simulink model "Controller"  (R2020a)
settings: Solver=FixedStepDiscrete  StartTime=0.0  StopTime=inf  FixedStep=Ts  RelTol=1e-3
values from neighbouring files (symbols this model uses):
  driver_decel = 4.0    (= 4)    [helperLFSetUp.m]
  FB_decel = 9.8    [helperLFSetUp.m]
  Fyf1 = zeros(1,57)    [FyfLookup05.m]
  headwayOffset = 3.7    [helperLFSetUp.m]
  m = 2272    [FyfLookup05.m]    (also in helperLFSetUp.m)
  max_dc = -10    [helperLFSetUp.m]
  PB1_decel = 3.8    [helperLFSetUp.m]
  PB2_decel = 5.3    [helperLFSetUp.m]
  posSelector = [1,0,0,0,0,0; 0,0,1,0,0,0]    [helperLFSetUp.m]
  PredictionHorizon = 30    [helperLFSetUp.m]
  PredictionHorizon1 = 60    [helperLFSetUp.m]
  SlipAngle1 = -SlipAngle1    [FyfLookup05.m]
  time_gap = 1.5    [helperLFSetUp.m]
  timeMargin = 0    [helperLFSetUp.m]
  timeToReact = 1.2    [helperLFSetUp.m]
  Ts = 0.1    [helperLFSetUp.m]
libraries: drivinglib x4, simulink x2, mpcadaslib x1, mpclib x1, simulink_extras x1
(part 1 of 2)
settings Model: Creator=The MathWorks, Inc.  LastModifiedBy=dekunw
settings DataIOCC: SaveOutput=off  SaveTime=off  ReturnWorkspaceOutputs=off
settings OptimizationCC: DefaultParameterBehavior=Inlined  DefaultUnderspecifiedDataType=single  EnhancedBackFolding=on  PassReuseOutputArgsAs=Individual arguments  ZeroExternalMemoryAtStartup=off  ZeroInternalMemoryAtStartup=off  OptimizeBlockOrder=speed  DifferentSizesBufferReuse=on  OptimizationCustomize=off  EfficientTunableParamExpr=on
settings DebuggingCC: ParameterPrecisionLossMsg=none  ParameterTunabilityLossMsg=error  PregeneratedLibrarySubsystemCodeDiagnostic=none  ArithmeticOperatorsInVariantConditions=warning
settings HardwareCC: ProdLongLongMode=on
settings SFSimCC: SimUseLocalCustomCode=off  MATLABDynamicMemAlloc=off  CustomCodeUndefinedFunction=UseInterfaceOnly
settings RTWCC: SystemTargetFile=ert.tlc  TemplateMakefile=ert_default_tmf  GenerateReport=on  RTWUseLocalCustomCode=off  BuildConfiguration=Faster Runs  IncludeHyperlinkInReport=on  LaunchReport=on  TargetLang=C++  GenerateTraceInfo=on  GenerateTraceReport=on  GenerateTraceReportSl=on  GenerateTraceReportSf=on  GenerateTraceReportEml=on
settings CodeAppCC: ForceParamTrailComments=on  IgnoreCustomStorageClasses=off  MaxIdLength=63  OperatorAnnotations=on  SimulinkDataObjDesc=on  SFDataObjDesc=on  CustomSymbolStrFcn=$N$M$F  InsertBlockDesc=on
settings ERTTargetCC: TargetLangStandard=C++03 (ISO)  GenerateSampleERTMain=on  MultiInstanceERTCode=on  CodeInterfacePackaging=C++ class  InlinedParameterPlacement=NonHierarchical  RootIOFormat=Structure reference  ERTCustomFileTemplate=example_file_process.tlc

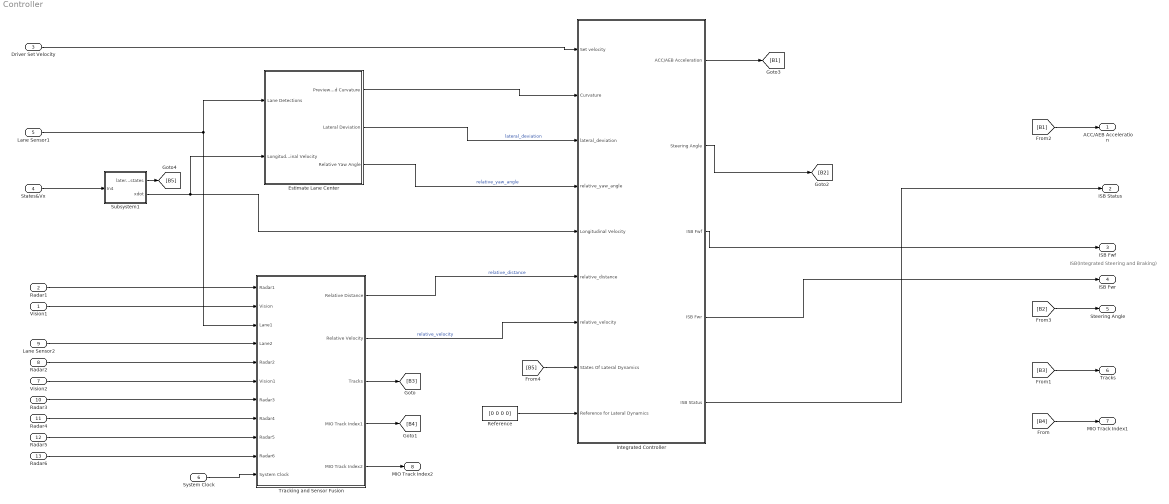
== system Controller ==
  note: ISB(Integrated Steering and Braking)
  Vision1 : Inport  OutDataTypeStr=Bus: BusVision  PortDimensions=[1 1]  BusOutputAsStruct=on
  Radar1 : Inport  Port=2  OutDataTypeStr=Bus: BusRadar  PortDimensions=[1 1]  BusOutputAsStruct=on
  Driver Set Velocity : Inport  Port=3
  States&Vx : Inport  Port=4  OutDataTypeStr=double  Unit=m/s
  Lane Sensor1 : Inport  Port=5  OutDataTypeStr=Bus: LaneSensor  PortDimensions=[1 1]
  System Clock : Inport  Port=6  OutDataTypeStr=double  PortDimensions=[1 1]
  Vision2 : Inport  Port=7  OutDataTypeStr=Bus: BusVision  PortDimensions=[1 1]  BusOutputAsStruct=on
  Radar2 : Inport  Port=8  OutDataTypeStr=Bus: BusRadar  PortDimensions=[1 1]  BusOutputAsStruct=on
  Lane Sensor2 : Inport  Port=9  OutDataTypeStr=Bus: LaneSensor  PortDimensions=[1 1]
  Radar3 : Inport  Port=10  OutDataTypeStr=Bus: BusRadar  PortDimensions=[1 1]  BusOutputAsStruct=on
  Radar4 : Inport  Port=11  OutDataTypeStr=Bus: BusRadar  PortDimensions=[1 1]  BusOutputAsStruct=on
  Radar5 : Inport  Port=12  OutDataTypeStr=Bus: BusRadar  PortDimensions=[1 1]  BusOutputAsStruct=on
  Radar6 : Inport  Port=13  OutDataTypeStr=Bus: BusRadar  PortDimensions=[1 1]  BusOutputAsStruct=on
  Estimate Lane Center : Subsystem  TreatAsAtomicUnit=on  VariantControl=v2
      settings: RTWFileNameOpts=Use function name
  Integrated Controller : Subsystem
  Reference : Constant  Value=[0 0 0 0]
  Subsystem1 : Subsystem
  Tracking and Sensor Fusion : Subsystem  TreatAsAtomicUnit=on
      settings: RTWFileNameOpts=Use function name
  ACC/AEB Acceleration : Outport  PortDimensions=1  VectorParamsAs1DForOutWhenUnconnected=off
  ISB Status : Outport  Port=2  PortDimensions=1  VectorParamsAs1DForOutWhenUnconnected=off
  ISB Fwf : Outport  Port=3  VectorParamsAs1DForOutWhenUnconnected=off
  ISB Fwr : Outport  Port=4  VectorParamsAs1DForOutWhenUnconnected=off
  Steering Angle : Outport  Port=5  PortDimensions=1  VectorParamsAs1DForOutWhenUnconnected=off
  Tracks : Outport  Port=6  OutDataTypeStr=Bus: BusMultiObjectTracker1  PortDimensions=[1 1]  VectorParamsAs1DForOutWhenUnconnected=off  BusOutputAsStruct=on
  MIO Track Index1 : Outport  Port=7  PortDimensions=1  VectorParamsAs1DForOutWhenUnconnected=off  BusOutputAsStruct=on
  MIO Track Index2 : Outport  Port=8  PortDimensions=1  VectorParamsAs1DForOutWhenUnconnected=off  BusOutputAsStruct=on
  wires:
  Lane Sensor1/1 -> Tracking and Sensor Fusion/3(Lane1), Estimate Lane Center/1(Lane Detections)
  Vision1/1 -> Tracking and Sensor Fusion/2(Vision)
  Radar1/1 -> Tracking and Sensor Fusion/1(Radar1)
  System Clock/1 -> Tracking and Sensor Fusion/11(System Clock)
  Estimate Lane Center/1(Previewed Curvature) -> Integrated Controller/2(Curvature)
  Estimate Lane Center/2(Lateral Deviation) -> Integrated Controller/3(lateral_deviation)  "lateral_deviation"
  Estimate Lane Center/3(Relative Yaw Angle) -> Integrated Controller/4(relative_yaw_angle)  "relative_yaw_angle"
  Tracking and Sensor Fusion/1(Relative Distance) -> Integrated Controller/6(relative_distance)  "relative_distance"
  Tracking and Sensor Fusion/2(Relative Velocity) -> Integrated Controller/7(relative_velocity)  "relative_velocity"
  Driver Set Velocity/1 -> Integrated Controller/1(Set velocity)
  Tracking and Sensor Fusion/3(Tracks) -> [B3]
  Tracking and Sensor Fusion/4(MIO Track Index1) -> [B4]
  [B4] -> MIO Track Index1/1
  [B3] -> Tracks/1
  Integrated Controller/2(Steering Angle) -> [B2]
  [B1] -> ACC/AEB Acceleration/1
  States&Vx/1 -> Subsystem1/1(In4)
  Subsystem1/1(lateral states) -> [B5]
  [B5] -> Integrated Controller/8(States Of Lateral Dynamics)
  Reference/1 -> Integrated Controller/9(Reference for Lateral Dynamics)
  Subsystem1/2(xdot) -> Integrated Controller/5(Longitudinal Velocity), Estimate Lane Center/2(Longitudinal Velocity)
  Integrated Controller/1(ACC/AEB Acceleration) -> [B1]
  Integrated Controller/3(ISB Fwf) -> ISB Fwf/1
  Integrated Controller/5(ISB Status) -> ISB Status/1
  Integrated Controller/4(ISB Fwr) -> ISB Fwr/1
  [B2] -> Steering Angle/1
  Lane Sensor2/1 -> Tracking and Sensor Fusion/4(Lane2)
  Radar2/1 -> Tracking and Sensor Fusion/5(Radar2)
  Vision2/1 -> Tracking and Sensor Fusion/6(Vision1)
  Radar3/1 -> Tracking and Sensor Fusion/7(Radar3)
  Radar4/1 -> Tracking and Sensor Fusion/8(Radar4)
  Radar5/1 -> Tracking and Sensor Fusion/9(Radar5)
  Radar6/1 -> Tracking and Sensor Fusion/10(Radar6)
  Tracking and Sensor Fusion/5(MIO Track Index2) -> MIO Track Index2/1

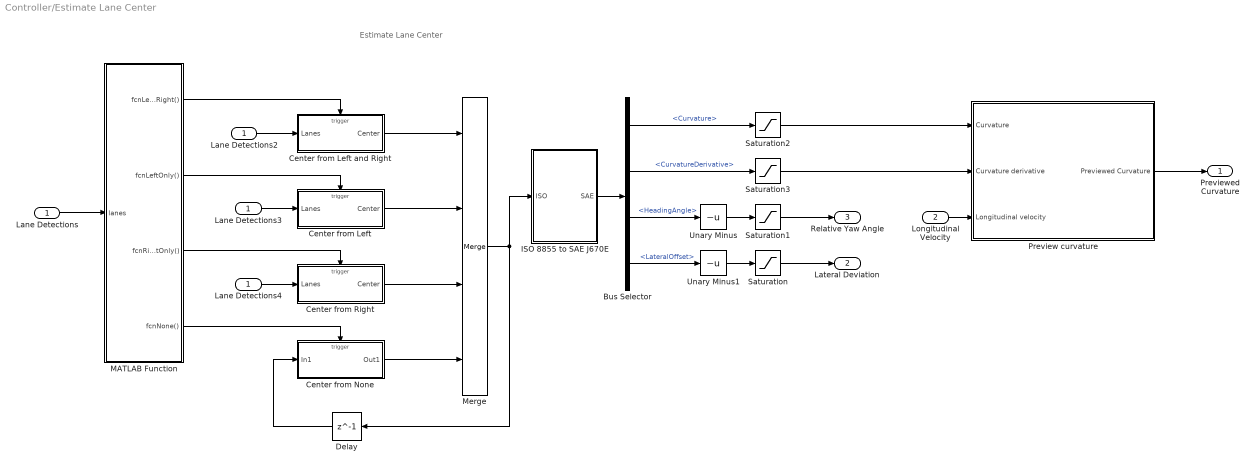
== system Controller/Estimate Lane Center ==
  note: Estimate Lane Center
  Lane Detections : Inport
  Longitudinal Velocity : Inport  Port=2
  Bus Selector : BusSelector  OutputSignals=Curvature,CurvatureDerivative,HeadingAngle,LateralOffset
  Center from Left : Subsystem  TreatAsAtomicUnit=on
  Center from Left and Right : Subsystem  TreatAsAtomicUnit=on
  Center from None : Subsystem  TreatAsAtomicUnit=on
  Center from Right : Subsystem  TreatAsAtomicUnit=on
  Delay : Delay  DelayLength=1
  ISO 8855 to SAE J670E : Subsystem
  Lane Detections2 : InportShadow
  Lane Detections3 : InportShadow
  Lane Detections4 : InportShadow
  MATLAB Function : MATLAB Function  TreatAsAtomicUnit=on
  Merge : Merge  Inputs=4
  Preview curvature : Subsystem
  Saturation : Saturate
  Saturation1 : Saturate  UpperLimit=0.6  LowerLimit=-0.6
  Saturation2 : Saturate  UpperLimit=0.15  LowerLimit=-0.15
  Saturation3 : Saturate  UpperLimit=0.06  LowerLimit=-0.06
  Unary Minus : UnaryMinus
  Unary Minus1 : UnaryMinus
  Previewed Curvature : Outport  VectorParamsAs1DForOutWhenUnconnected=off
  Lateral Deviation : Outport  Port=2  VectorParamsAs1DForOutWhenUnconnected=off
  Relative Yaw Angle : Outport  Port=3  VectorParamsAs1DForOutWhenUnconnected=off
  wires:
  Center from Right/1(Center) -> Merge/3
  Lane Detections3/1 -> Center from Left/1(Lanes)
  Lane Detections4/1 -> Center from Right/1(Lanes)
  MATLAB Function/2(fcnLeftOnly()) -> Center from Left/Trigger
  Center from None/1(Out1) -> Merge/4
  MATLAB Function/1(fcnLeftAndRight()) -> Center from Left and Right/Trigger
  Delay/1 -> Center from None/1(In1)
  Center from Left and Right/1(Center) -> Merge/1
  Lane Detections/1 -> MATLAB Function/1(lanes)
  Lane Detections2/1 -> Center from Left and Right/1(Lanes)
  MATLAB Function/3(fcnRightOnly()) -> Center from Right/Trigger
  MATLAB Function/4(fcnNone()) -> Center from None/Trigger
  Center from Left/1(Center) -> Merge/2
  Merge/1 -> ISO 8855 to SAE J670E/1(ISO), Delay/1
  Saturation3/1 -> Preview curvature/2(Curvature derivative)
  Saturation2/1 -> Preview curvature/1(Curvature)
  Saturation1/1 -> Relative Yaw Angle/1
  Saturation/1 -> Lateral Deviation/1
  Unary Minus/1 -> Saturation1/1
  Preview curvature/1(Previewed Curvature) -> Previewed Curvature/1
  Longitudinal Velocity/1 -> Preview curvature/3(Longitudinal velocity)
  Bus Selector/2 -> Saturation3/1  "<CurvatureDerivative>"
  Bus Selector/1 -> Saturation2/1  "<Curvature>"
  Unary Minus1/1 -> Saturation/1
  Bus Selector/4 -> Unary Minus1/1  "<LateralOffset>"
  Bus Selector/3 -> Unary Minus/1  "<HeadingAngle>"
  ISO 8855 to SAE J670E/1(SAE) -> Bus Selector/1

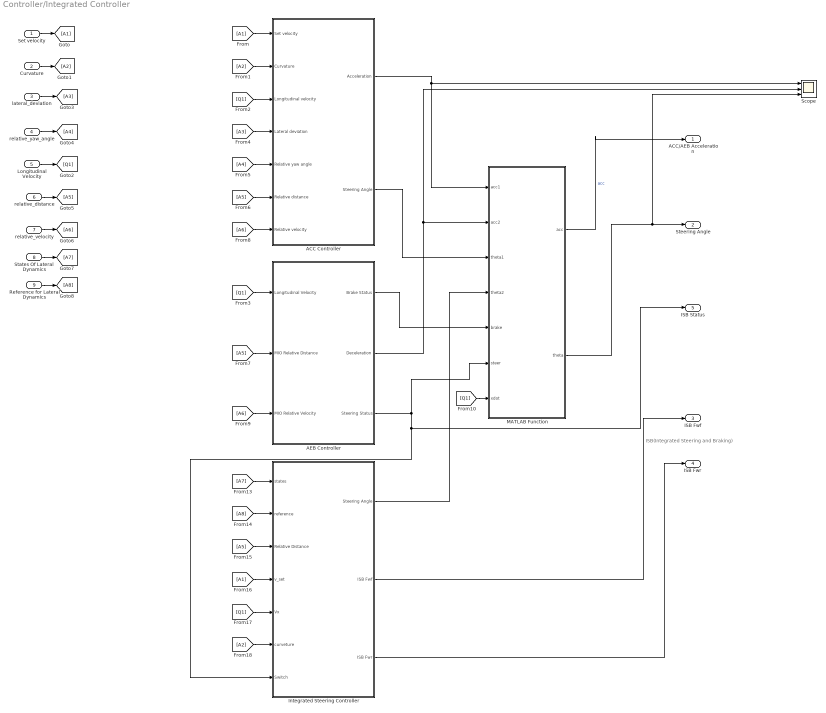
== system Controller/Integrated Controller ==
  note: ISB(Integrated Steering and Braking)
  Set velocity : Inport
  Curvature : Inport  Port=2
  lateral_deviation : Inport  Port=3
  relative_yaw_angle : Inport  Port=4
  Longitudinal Velocity : Inport  Port=5
  relative_distance : Inport  Port=6
  relative_velocity : Inport  Port=7
  States Of Lateral Dynamics : Inport  Port=8
  Reference for Lateral Dynamics : Inport  Port=9
  ACC Controller : Subsystem
  AEB Controller : Subsystem
  Integrated Steering Controller : Subsystem
  MATLAB Function : MATLAB Function  TreatAsAtomicUnit=on
  Scope : Scope  NumInputPorts=3
  ACC/AEB Acceleration : Outport
  Steering Angle : Outport  Port=2
  ISB Fwf : Outport  Port=3
  ISB Fwr : Outport  Port=4
  ISB Status : Outport  Port=5
  wires:
  Set velocity/1 -> [A1]
  [A1] -> ACC Controller/1(Set velocity)
  Curvature/1 -> [A2]
  [A2] -> ACC Controller/2(Curvature)
  [Q1] -> ACC Controller/3(Longitudinal velocity)
  [Q1] -> AEB Controller/1(Longitudinal Velocity)
  lateral_deviation/1 -> [A3]
  [A3] -> ACC Controller/4(Lateral deviation)
  relative_yaw_angle/1 -> [A4]
  [A4] -> ACC Controller/5(Relative yaw angle)
  relative_distance/1 -> [A5]
  [A5] -> ACC Controller/6(Relative distance)
  [A5] -> AEB Controller/2(MIO Relative Distance)
  relative_velocity/1 -> [A6]
  [A6] -> ACC Controller/7(Relative velocity)
  [A6] -> AEB Controller/3(MIO Relative Velocity)
  States Of Lateral Dynamics/1 -> [A7]
  Reference for Lateral Dynamics/1 -> [A8]
  [A7] -> Integrated Steering Controller/1(states)
  [A8] -> Integrated Steering Controller/2(reference)
  [A5] -> Integrated Steering Controller/3(Relative Distance)
  [A1] -> Integrated Steering Controller/4(v_set)
  [Q1] -> Integrated Steering Controller/5(Vx)
  [A2] -> Integrated Steering Controller/6(curveture)
  Longitudinal Velocity/1 -> [Q1]
  AEB Controller/3(Steering Status) -> MATLAB Function/6(steer), Integrated Steering Controller/7(Switch), ISB Status/1
  ACC Controller/1(Acceleration) -> MATLAB Function/1(acc1), Scope/1
  AEB Controller/2(Deceleration) -> Scope/2, MATLAB Function/2(acc2)
  AEB Controller/1(Brake Status) -> MATLAB Function/5(brake)
  ACC Controller/2(Steering Angle) -> MATLAB Function/3(theta1)
  Integrated Steering Controller/1(Steering Angle) -> MATLAB Function/4(theta2)
  [Q1] -> MATLAB Function/7(xdot)
  MATLAB Function/1(acc) -> ACC/AEB Acceleration/1  "acc"
  MATLAB Function/2(theta) -> Scope/3, Steering Angle/1
  Integrated Steering Controller/2(ISB Fwf) -> ISB Fwf/1
  Integrated Steering Controller/3(ISB Fwr) -> ISB Fwr/1

== system Controller/Subsystem1 ==
  In4 : Inport
  Demux : Demux  Outputs=5
  Mux : Mux
  lateral states : Outport
  xdot : Outport  Port=2
  wires:
  In4/1 -> Demux/1
  Demux/1 -> Mux/1
  Demux/2 -> Mux/2
  Demux/3 -> Mux/3
  Demux/5 -> xdot/1
  Demux/4 -> Mux/4
  Mux/1 -> lateral states/1

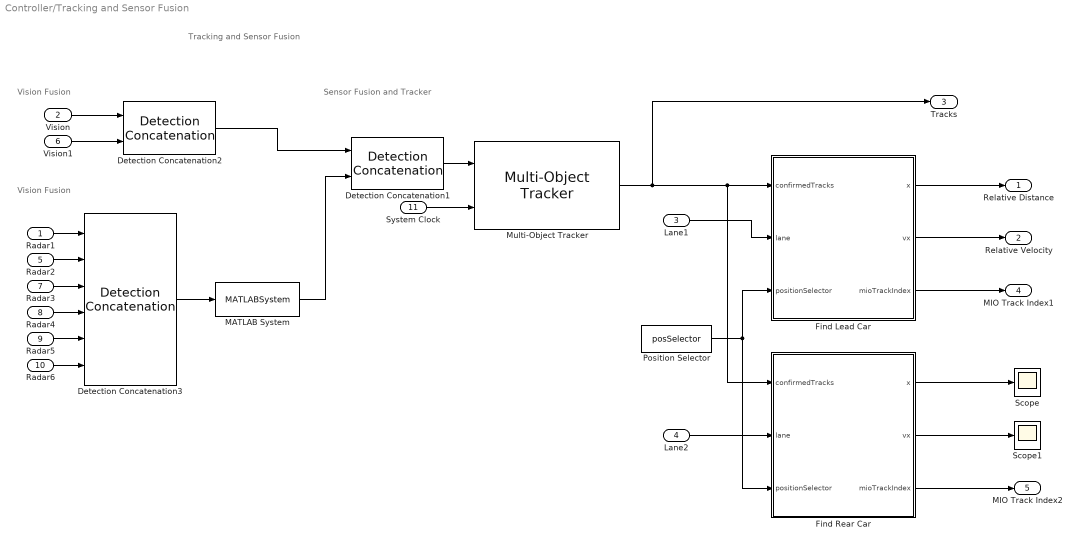
== system Controller/Tracking and Sensor Fusion ==
  note: Tracking and Sensor Fusion
  note: Vision Fusion
  note: Sensor Fusion and Tracker
  note: Vision Fusion
  Radar1 : Inport  OutDataTypeStr=Bus: BusRadar  PortDimensions=[1 1]  BusOutputAsStruct=on
  Vision : Inport  Port=2  OutDataTypeStr=Bus: BusVision  PortDimensions=[1 1]  BusOutputAsStruct=on
  Lane1 : Inport  Port=3  OutDataTypeStr=Bus: LaneSensor  BusOutputAsStruct=on
  Lane2 : Inport  Port=4  OutDataTypeStr=Bus: LaneSensor  BusOutputAsStruct=on
  Radar2 : Inport  Port=5  OutDataTypeStr=Bus: BusRadar  PortDimensions=[1 1]  BusOutputAsStruct=on
  Vision1 : Inport  Port=6  OutDataTypeStr=Bus: BusVision  PortDimensions=[1 1]  BusOutputAsStruct=on
  Radar3 : Inport  Port=7  OutDataTypeStr=Bus: BusRadar  PortDimensions=[1 1]  BusOutputAsStruct=on
  Radar4 : Inport  Port=8  OutDataTypeStr=Bus: BusRadar  PortDimensions=[1 1]  BusOutputAsStruct=on
  Radar5 : Inport  Port=9  OutDataTypeStr=Bus: BusRadar  PortDimensions=[1 1]  BusOutputAsStruct=on
  Radar6 : Inport  Port=10  OutDataTypeStr=Bus: BusRadar  PortDimensions=[1 1]  BusOutputAsStruct=on
  System Clock : Inport  Port=11  OutDataTypeStr=double  PortDimensions=[1 1]
  Detection Concatenation1 : drivinglib/Detection Concatenation  NumInputs=2  BusNameSource=Auto  BusName=BusDetectionConcatenation1  SimulateUsing=Interpreted execution
      settings: SourceProductBaseCode=DR
  Detection Concatenation2 : drivinglib/Detection Concatenation  NumInputs=2  BusNameSource=Auto  BusName=BusDetectionConcatenation1  SimulateUsing=Interpreted execution
      settings: SourceProductBaseCode=DR
  Detection Concatenation3 : drivinglib/Detection Concatenation  NumInputs=6  BusNameSource=Auto  BusName=BusDetectionConcatenation1  SimulateUsing=Interpreted execution
      settings: SourceProductBaseCode=DR
  Find Lead Car : MATLAB Function  TreatAsAtomicUnit=on
  Find Rear Car : MATLAB Function  TreatAsAtomicUnit=on
  MATLAB System : MATLABSystem  System=helperClusterDetections  ClusterSize=clusterSize  BusNameSource=Auto  BusName=BusClusterDetections  SimulateUsing=Interpreted execution
      mask Type: helperClusterDetections
      mask Display:
      | disp(['Detection' char(10) 'Clustering']);
      | port_label('input',1,'In');
      | port_label('output',1,'Out');
  Multi-Object Tracker : drivinglib/Multi-Object Tracker  TrackerIndex=uint32( 0 )  FilterInitializationFcn=initcvekf  AssignmentThreshold=assigThresh  ConfirmationThreshold=[ 2, 3 ]  DeletionThreshold=[ 5, 5 ]  MaxNumTracks=numTracks  MaxNumSensors=numSensors  StateParams=struct  TimeInputSource=Input port  HasCostMatrixInput=off  HasDetectableTrackIDsInput=off  BusNameSource=Property  BusName=BusMultiObjectTracker1  TentativeTracksOutputPort=off  AllTracksOutputPort=off  SimulateUsing=Interpreted execution
      settings: SourceProductBaseCode=DR
  Position Selector : Constant  Value=posSelector
  Scope : Scope
  Scope1 : Scope
  Relative Distance : Outport  VectorParamsAs1DForOutWhenUnconnected=off
  Relative Velocity : Outport  Port=2  VectorParamsAs1DForOutWhenUnconnected=off
  Tracks : Outport  Port=3  OutDataTypeStr=Bus:BusMultiObjectTracker1  PortDimensions=[1 1]  VectorParamsAs1DForOutWhenUnconnected=off  BusOutputAsStruct=on
  MIO Track Index1 : Outport  Port=4  VectorParamsAs1DForOutWhenUnconnected=off
  MIO Track Index2 : Outport  Port=5  VectorParamsAs1DForOutWhenUnconnected=off
  wires:
  Position Selector/1 -> Find Lead Car/3(positionSelector), Find Rear Car/3(positionSelector)
  Lane1/1 -> Find Lead Car/2(lane)
  Detection Concatenation1/1 -> Multi-Object Tracker/1
  Multi-Object Tracker/1 -> Find Rear Car/1(confirmedTracks), Find Lead Car/1(confirmedTracks), Tracks/1
  Detection Concatenation3/1 -> MATLAB System/1
  System Clock/1 -> Multi-Object Tracker/2
  Detection Concatenation2/1 -> Detection Concatenation1/1
  MATLAB System/1 -> Detection Concatenation1/2
  Vision1/1 -> Detection Concatenation2/2
  Vision/1 -> Detection Concatenation2/1
  Radar1/1 -> Detection Concatenation3/1
  Radar2/1 -> Detection Concatenation3/2
  Radar6/1 -> Detection Concatenation3/6
  Radar5/1 -> Detection Concatenation3/5
  Radar4/1 -> Detection Concatenation3/4
  Radar3/1 -> Detection Concatenation3/3
  Find Lead Car/1(x) -> Relative Distance/1
  Find Lead Car/2(vx) -> Relative Velocity/1
  Find Lead Car/3(mioTrackIndex) -> MIO Track Index1/1
  Lane2/1 -> Find Rear Car/2(lane)
  Find Rear Car/1(x) -> Scope/1
  Find Rear Car/2(vx) -> Scope1/1
  Find Rear Car/3(mioTrackIndex) -> MIO Track Index2/1

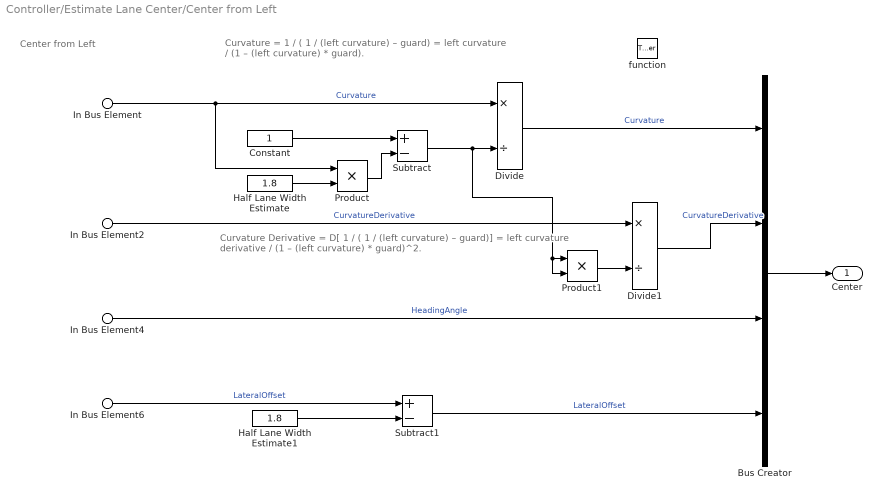
== system Controller/Estimate Lane Center/Center from Left ==
  note: Curvature Derivative
      | = D[ 1 / ( 1 / (left curvature) – guard)]
      | = left curvature derivative / (1 – (left curvature) * guard)^2.
  note: Center from Left
  note: Curvature
      | = 1 / ( 1 / (left curvature) – guard)
      | = left curvature / (1 – (left curvature) * guard).
  In Bus Element : Inport  PortName=Lanes  Element=Left.Curvature
  In Bus Element2 : Inport  PortName=Lanes  Element=Left.CurvatureDerivative
  In Bus Element4 : Inport  PortName=Lanes  Element=Left.HeadingAngle
  In Bus Element6 : Inport  PortName=Lanes  Element=Left.LateralOffset
  function : TriggerPort  TriggerType=function-call  VariantControl=Variant
  Bus Creator : BusCreator  Inputs=4
  Constant : Constant  OutDataTypeStr=Inherit: Inherit via back propagation
  Divide : Product  Inputs=*/
  Divide1 : Product  Inputs=*/
  Half Lane Width Estimate : Constant  Value=1.8  OutDataTypeStr=Inherit: Inherit via back propagation
  Half Lane Width Estimate1 : Constant  Value=1.8  OutDataTypeStr=Inherit: Inherit via back propagation
  Product : Product
  Product1 : Product
  Subtract : Sum  Inputs=+-
  Subtract1 : Sum  Inputs=+-
  Center : Outport  VectorParamsAs1DForOutWhenUnconnected=off
  wires:
  Product/1 -> Subtract/2
  Half Lane Width Estimate1/1 -> Subtract1/2
  In Bus Element6/1 -> Subtract1/1  "LateralOffset"
  Product1/1 -> Divide1/2
  In Bus Element2/1 -> Divide1/1  "CurvatureDerivative"
  Constant/1 -> Subtract/1
  Half Lane Width Estimate/1 -> Product/2
  Subtract/1 -> Divide/2, Product1/1, Product1/2
  In Bus Element/1 -> Divide/1, Product/1  "Curvature"
  Subtract1/1 -> Bus Creator/4  "LateralOffset"
  In Bus Element4/1 -> Bus Creator/3  "HeadingAngle"
  Divide/1 -> Bus Creator/1  "Curvature"
  Divide1/1 -> Bus Creator/2  "CurvatureDerivative"
  Bus Creator/1 -> Center/1

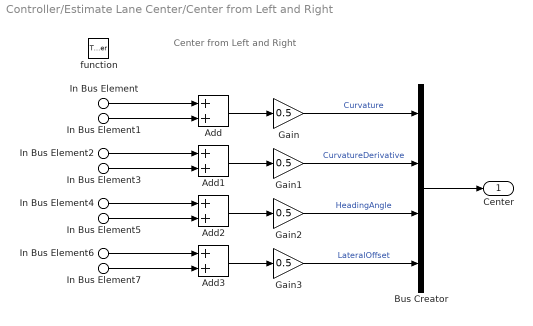
== system Controller/Estimate Lane Center/Center from Left and Right ==
  note: Center from Left and Right
  In Bus Element : Inport  PortName=Lanes  Element=Left.Curvature
  In Bus Element2 : Inport  PortName=Lanes  Element=Left.CurvatureDerivative
  In Bus Element4 : Inport  PortName=Lanes  Element=Left.HeadingAngle
  In Bus Element6 : Inport  PortName=Lanes  Element=Left.LateralOffset
  In Bus Element1 : Inport  PortName=Lanes  Element=Right.Curvature
  In Bus Element3 : Inport  PortName=Lanes  Element=Right.CurvatureDerivative
  In Bus Element5 : Inport  PortName=Lanes  Element=Right.HeadingAngle
  In Bus Element7 : Inport  PortName=Lanes  Element=Right.LateralOffset
  function : TriggerPort  TriggerType=function-call  VariantControl=Variant
  Add{,1..3} (4 alike) : Sum
  Bus Creator : BusCreator  Inputs=4
  Gain{,1..3} (4 alike) : Gain  Gain=0.5
  Center : Outport  VectorParamsAs1DForOutWhenUnconnected=off
  wires:
  In Bus Element6/1 -> Add3/1
  In Bus Element7/1 -> Add3/2
  In Bus Element5/1 -> Add2/2
  In Bus Element4/1 -> Add2/1
  In Bus Element3/1 -> Add1/2
  In Bus Element2/1 -> Add1/1
  In Bus Element1/1 -> Add/2
  In Bus Element/1 -> Add/1
  Bus Creator/1 -> Center/1
  Gain3/1 -> Bus Creator/4  "LateralOffset"
  Add3/1 -> Gain3/1
  Gain2/1 -> Bus Creator/3  "HeadingAngle"
  Add2/1 -> Gain2/1
  Gain1/1 -> Bus Creator/2  "CurvatureDerivative"
  Add1/1 -> Gain1/1
  Gain/1 -> Bus Creator/1  "Curvature"
  Add/1 -> Gain/1

== system Controller/Estimate Lane Center/Center from None ==
  In1 : Inport
  function : TriggerPort  TriggerType=function-call  VariantControl=Variant
  Out1 : Outport  VectorParamsAs1DForOutWhenUnconnected=off
  wires:
  In1/1 -> Out1/1

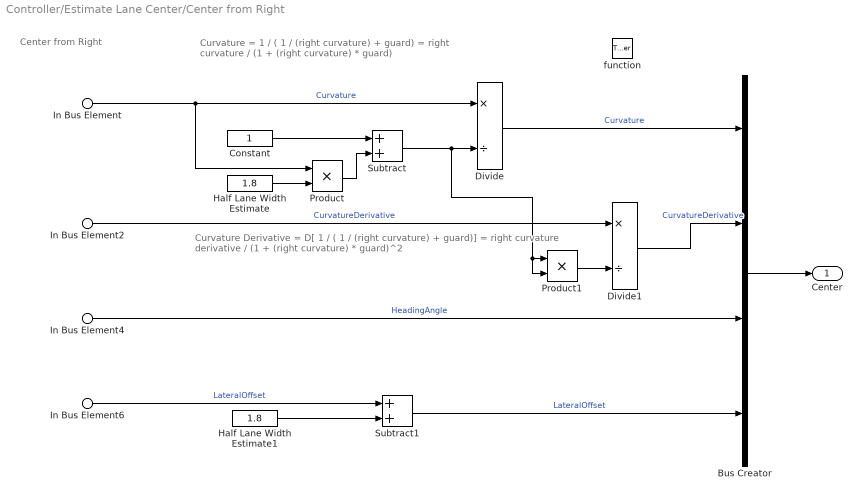
== system Controller/Estimate Lane Center/Center from Right ==
  note: Curvature Derivative
      | = D[ 1 / ( 1 / (right curvature) + guard)]
      | = right curvature derivative / (1 + (right curvature) * guard)^2
  note: Curvature
      | = 1 / ( 1 / (right curvature) + guard)
      | = right curvature / (1 + (right curvature) * guard)
  note: Center from Right
  In Bus Element : Inport  PortName=Lanes  Element=Right.Curvature
  In Bus Element2 : Inport  PortName=Lanes  Element=Right.CurvatureDerivative
  In Bus Element4 : Inport  PortName=Lanes  Element=Right.HeadingAngle
  In Bus Element6 : Inport  PortName=Lanes  Element=Right.LateralOffset
  function : TriggerPort  TriggerType=function-call  VariantControl=Variant
  Bus Creator : BusCreator  Inputs=4
  Constant : Constant  OutDataTypeStr=Inherit: Inherit via back propagation
  Divide : Product  Inputs=*/
  Divide1 : Product  Inputs=*/
  Half Lane Width Estimate : Constant  Value=1.8  OutDataTypeStr=Inherit: Inherit via back propagation
  Half Lane Width Estimate1 : Constant  Value=1.8  OutDataTypeStr=Inherit: Inherit via back propagation
  Product : Product
  Product1 : Product
  Subtract : Sum
  Subtract1 : Sum
  Center : Outport  VectorParamsAs1DForOutWhenUnconnected=off
  wires:
  Half Lane Width Estimate/1 -> Product/2
  Product/1 -> Subtract/2
  Constant/1 -> Subtract/1
  Subtract/1 -> Divide/2, Product1/1, Product1/2
  In Bus Element/1 -> Divide/1, Product/1  "Curvature"
  Bus Creator/1 -> Center/1
  Subtract1/1 -> Bus Creator/4  "LateralOffset"
  Divide/1 -> Bus Creator/1  "Curvature"
  In Bus Element6/1 -> Subtract1/1  "LateralOffset"
  Half Lane Width Estimate1/1 -> Subtract1/2
  In Bus Element4/1 -> Bus Creator/3  "HeadingAngle"
  Product1/1 -> Divide1/2
  Divide1/1 -> Bus Creator/2  "CurvatureDerivative"
  In Bus Element2/1 -> Divide1/1  "CurvatureDerivative"

== system Controller/Estimate Lane Center/ISO 8855 to SAE J670E ==
  note: positive Y is to the left in ISO 8855
      | positive Y is to the right in SAE J670E
  note: ISO 8855 to SAE J670E
  ISO : Inport
  Bus Creator : BusCreator  Inputs=4
  Bus Selector : BusSelector  OutputSignals=CurvatureDerivative,Curvature,HeadingAngle,LateralOffset
  Signal Specification : SignalSpecification  Unit=1/m^2
  Signal Specification1 : SignalSpecification  Unit=1/m
  Signal Specification2 : SignalSpecification  Unit=rad
  Signal Specification3 : SignalSpecification  Unit=m
  Unary Minus{,1..3} (4 alike) : UnaryMinus
  SAE : Outport  VectorParamsAs1DForOutWhenUnconnected=off
  wires:
  ISO/1 -> Bus Selector/1
  Bus Selector/2 -> Unary Minus/1  "<Curvature>"
  Bus Selector/1 -> Unary Minus1/1  "<CurvatureDerivative>"
  Bus Selector/3 -> Unary Minus2/1  "<HeadingAngle>"
  Bus Selector/4 -> Unary Minus3/1  "<LateralOffset>"
  Bus Creator/1 -> SAE/1
  Signal Specification/1 -> Bus Creator/2  "Curvature"
  Unary Minus1/1 -> Signal Specification1/1
  Unary Minus2/1 -> Signal Specification2/1
  Unary Minus3/1 -> Signal Specification3/1
  Unary Minus/1 -> Signal Specification/1
  Signal Specification1/1 -> Bus Creator/1  "CurvatureDerivative"
  Signal Specification2/1 -> Bus Creator/3  "HeadingAngle"
  Signal Specification3/1 -> Bus Creator/4  "LateralOffset"

== system Controller/Estimate Lane Center/Preview curvature ==
  Curvature : Inport
  Curvature derivative : Inport  Port=2
  Longitudinal velocity : Inport  Port=3
  Gain : Gain  Gain=[0:Ts:PredictionHorizon*Ts]'
  Product : Product
  Sum : Sum
  Previewed Curvature : Outport  VectorParamsAs1DForOutWhenUnconnected=off
  wires:
  Sum/1 -> Previewed Curvature/1
  Curvature/1 -> Sum/1
  Gain/1 -> Sum/2
  Product/1 -> Gain/1
  Longitudinal velocity/1 -> Product/2
  Curvature derivative/1 -> Product/1

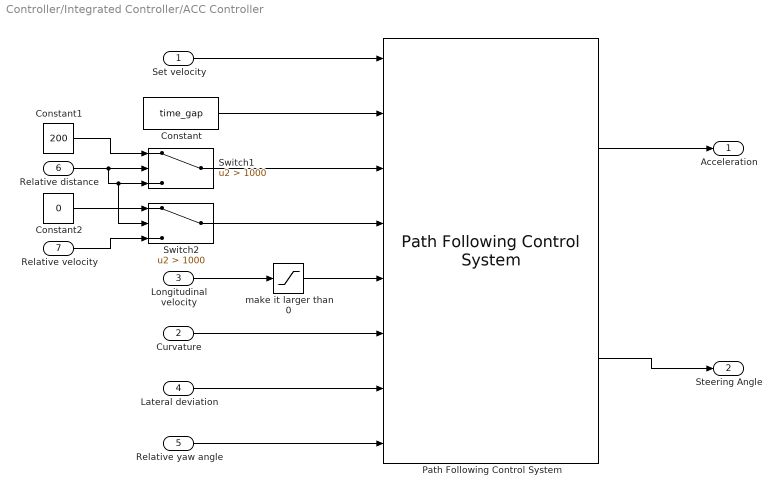
== system Controller/Integrated Controller/ACC Controller ==
  Set velocity : Inport
  Curvature : Inport  Port=2
  Longitudinal velocity : Inport  Port=3
  Lateral deviation : Inport  Port=4
  Relative yaw angle : Inport  Port=5
  Relative distance : Inport  Port=6
  Relative velocity : Inport  Port=7
  Constant : Constant  Value=time_gap
  Constant1 : Constant  Value=200
  Constant2 : Constant  Value=0
  Path Following Control System : mpcadaslib/Path Following Control System  VariantControl=Variant2  ModelType=Use vehicle parameters  VehicleMass=m  VehicleYawInertia=Iz  LengthToFront=lf  LengthToRear=lr  FrontTireStiffness=Cf  RearTireStiffness=Cr  AccelTimeConstant=tau  EgoModelMatrixA=[-2,zeros(1,3);1,zeros(1,3);zeros(1,2),-4.4021,-12.4603;zeros(1,2),1.3913,-5.1868]  EgoModelMatrixB=[2,zeros(1,3);zeros(1,2),24.1270,15.8609]'  EgoModelMatrixC=[zeros(3,1),eye(3)]  InitialLongVel=v0_ego  TransportLag=Ts  spaceCtrl=on  DefaultSpacing=default_spacing  MinSteering=min_steer  umin_ext=off  MaxSteering=max_steer  umax_ext=off  MinAcceleration=min_ac  amin_ext=off  MaxAcceleration=max_ac  amax_ext=off  Ts=Ts  PredictionHorizon=PredictionHorizon  ControlHorizon=2  LongWeight=0.1  LateralWeight=1  AccelRateWeight=0.1  SteerRateWeight=0.1  suboptimal=off  maxiter=10  datatypeopt=double  optmode=off  trackmode=off
      settings: SourceProductBaseCode=MP
  Switch1 : Switch  Criteria=u2 > Threshold  Threshold=1000
  Switch2 : Switch  Criteria=u2 > Threshold  Threshold=1000
  make it larger than 0 : Saturate  UpperLimit=200  LowerLimit=1e-6
  Acceleration : Outport  VectorParamsAs1DForOutWhenUnconnected=off
  Steering Angle : Outport  Port=2  VectorParamsAs1DForOutWhenUnconnected=off
  wires:
  Set velocity/1 -> Path Following Control System/1
  Curvature/1 -> Path Following Control System/6
  Longitudinal velocity/1 -> make it larger than 0/1
  Lateral deviation/1 -> Path Following Control System/7
  Relative yaw angle/1 -> Path Following Control System/8
  Constant/1 -> Path Following Control System/2
  Relative distance/1 -> Switch2/2, Switch1/3, Switch1/2
  Constant1/1 -> Switch1/1
  Switch1/1 -> Path Following Control System/3
  Relative velocity/1 -> Switch2/3
  Constant2/1 -> Switch2/1
  Switch2/1 -> Path Following Control System/4
  Path Following Control System/2 -> Steering Angle/1
  Path Following Control System/1 -> Acceleration/1
  make it larger than 0/1 -> Path Following Control System/5

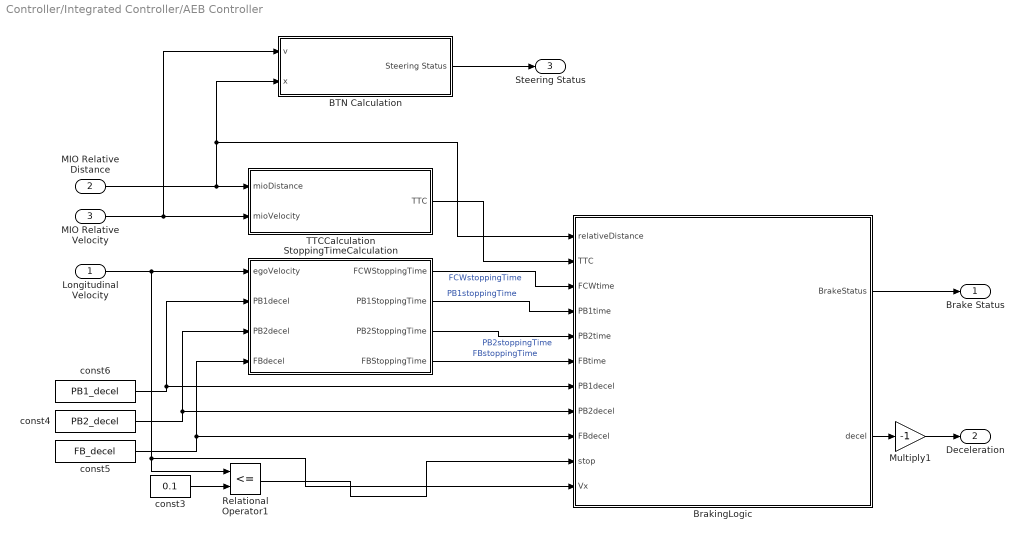
== system Controller/Integrated Controller/AEB Controller ==
  Longitudinal Velocity : Inport
  MIO Relative Distance : Inport  Port=2
  MIO Relative Velocity : Inport  Port=3
  BTN Calculation : Subsystem
  BrakingLogic : Stateflow chart  TreatAsAtomicUnit=on
  Multiply1 : Gain  Gain=-1
  Relational Operator1 : RelationalOperator  Operator=<=  OutDataTypeStr=boolean  RndMeth=Simplest
  StoppingTimeCalculation : Subsystem
  TTCCalculation : Subsystem
  const3 : Constant  Value=0.1  SampleTime=-1
  const4 : Constant  Value=PB2_decel  SampleTime=-1
  const5 : Constant  Value=FB_decel  SampleTime=-1
  const6 : Constant  Value=PB1_decel  SampleTime=-1
  Brake Status : Outport  VectorParamsAs1DForOutWhenUnconnected=off
  Deceleration : Outport  Port=2  VectorParamsAs1DForOutWhenUnconnected=off
  Steering Status : Outport  Port=3  VectorParamsAs1DForOutWhenUnconnected=off
  wires:
  Longitudinal Velocity/1 -> StoppingTimeCalculation/1(egoVelocity), BrakingLogic/11(Vx), Relational Operator1/1
  const4/1 -> BrakingLogic/8(PB2decel), StoppingTimeCalculation/3(PB2decel)
  const5/1 -> StoppingTimeCalculation/4(FBdecel), BrakingLogic/9(FBdecel)
  BrakingLogic/1(BrakeStatus) -> Brake Status/1
  const3/1 -> Relational Operator1/2
  Relational Operator1/1 -> BrakingLogic/10(stop)
  const6/1 -> BrakingLogic/7(PB1decel), StoppingTimeCalculation/2(PB1decel)
  StoppingTimeCalculation/3(PB2StoppingTime) -> BrakingLogic/5(PB2time)  "PB2stoppingTime"
  StoppingTimeCalculation/2(PB1StoppingTime) -> BrakingLogic/4(PB1time)  "PB1stoppingTime"
  StoppingTimeCalculation/4(FBStoppingTime) -> BrakingLogic/6(FBtime)  "FBstoppingTime"
  StoppingTimeCalculation/1(FCWStoppingTime) -> BrakingLogic/3(FCWtime)  "FCWstoppingTime"
  MIO Relative Distance/1 -> BTN Calculation/2(x), BrakingLogic/1(relativeDistance), TTCCalculation/1(mioDistance)
  MIO Relative Velocity/1 -> BTN Calculation/1(v), TTCCalculation/2(mioVelocity)
  TTCCalculation/1(TTC) -> BrakingLogic/2(TTC)
  BrakingLogic/2(decel) -> Multiply1/1
  Multiply1/1 -> Deceleration/1
  BTN Calculation/1(Steering Status) -> Steering Status/1

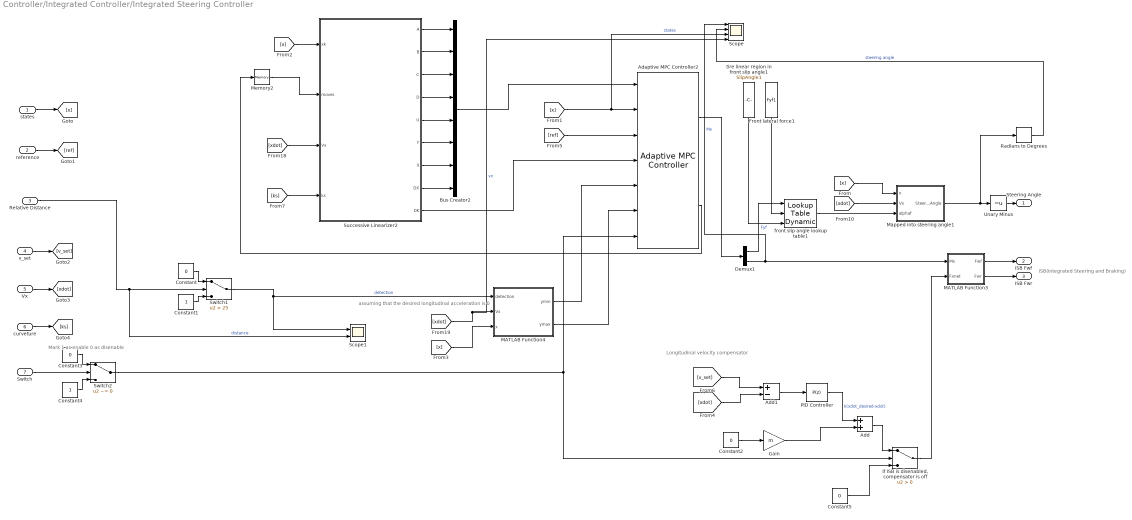
== system Controller/Integrated Controller/Integrated Steering Controller ==
  note: Longitudinal velocity compensator
  note: Mark 1 as enable 0 as disenable
  note: ISB(Integrated Steering and Braking)
  note: assuming that the desired longitudinal acceleration is 0
  states : Inport
  reference : Inport  Port=2
  Relative Distance : Inport  Port=3
  v_set : Inport  Port=4
  Vx : Inport  Port=5
  curveture : Inport  Port=6
  Switch : Inport  Port=7
  Adaptive MPC Controller2 : mpclib/Adaptive MPC Controller  SCDEnableBlockLinearizationSpecification=on  mpcobj=mpc008  enable_value=0  updateMPCinCallerWorkspace=on  md_inport=on  mv_inport=off  uref_inport=off  return_cost=off  return_mvseq=on  return_qpstatus=off  return_xseq=off  return_state=off  return_ovseq=off  state_inport=off  isltv_plant=on  umin_inport=off  umax_inport=off  ymin_inport=on  ymax_inport=on  cc_inport=off  ywt_inport=off  uwt_inport=off  duwt_inport=off  rhoeps_inport=off  pm_inport=off  MaximumP=10  HorizonChoice=FixedHorizon  BlockDataType=double  SampleTimeInherited=off  switch_inport=on
  Add : Sum
  Add1 : Sum  Inputs=+-
  Bus Creator2 : BusCreator  Inputs=8
  Constant{,2..3,5} (4 alike) : Constant  Value=0
  Constant1 : Constant
  Constant4 : Constant
  Demux1 : Demux  Outputs=2
  Front lateral force1 : Constant  Value=Fyf1
  Gain : Gain  Gain=m
  "If ISB is disenabled, compensator is off" : Switch  Criteria=u2 > Threshold
  MATLAB Function3 : MATLAB Function  TreatAsAtomicUnit=on
  MATLAB Function4 : MATLAB Function  TreatAsAtomicUnit=on
  Mapped into steering angle1 : MATLAB Function  TreatAsAtomicUnit=on
  Memory2 : Memory
  PID Controller : simulink/Continuous/PID Controller  Controller=P  Form=Parallel  TimeDomain=Discrete-time  UseExternalTs=off  SampleTime=-1  IntegratorMethod=Forward Euler  FilterMethod=Forward Euler  ControllerParametersSource=internal  P=5000  I=1  D=0  UseFilter=on  N=100  TunerSelectOption=Transfer Function Based (PID Tuner App)  InitialConditionSource=internal  InitialConditionForIntegrator=0  InitialConditionForFilter=0  DifferentiatorICPrevScaledInput=0  ExternalReset=none  TrackingMode=off  Kt=1  LimitOutput=off  UpperSaturationLimit=inf  LowerSaturationLimit=-inf  LinearizeAsGain=on  AntiWindupMode=none  Kb=1  POutMin=[]  POutMax=[]  IOutMin=[]  IOutMax=[]  DOutMin=[]  DOutMax=[]  NOutMin=[]  NOutMax=[]  SumOutMin=[]  SumOutMax=[]  SaturationOutMin=[]  SaturationOutMax=[]  PParamMin=[]  PParamMax=[]  IParamMin=[]  IParamMax=[]  DParamMin=[]  DParamMax=[]  NParamMin=[]  NParamMax=[]  KbParamMin=[]  KbParamMax=[]  KtParamMin=[]  KtParamMax=[]  KbOutMin=[]  KbOutMax=[]  KtOutMin=[]  KtOutMax=[]  IntegratorOutMin=[]  IntegratorOutMax=[]  FilterOutMin=[]  FilterOutMax=[]  SumI1OutMin=[]  SumI1OutMax=[]  SumI2OutMin=[]  SumI2OutMax=[]  SumI3OutMin=[]  SumI3OutMax=[]  SumI4OutMin=[]  SumI4OutMax=[]  SumDOutMin=[]  SumDOutMax=[]  DifferentiatorOutMin=[]  DifferentiatorOutMax=[]  FilterDiffOutCoefMin=[]  FilterDiffOutCoefMax=[]  ReciprocalOutMin=[]  ReciprocalOutMax=[]  SumDenOutMin=[]  SumDenOutMax=[]  SumNumOutMin=[]  SumNumOutMax=[]  DivideOutMin=[]  DivideOutMax=[]  UdiffTsProdOutMin=[]  UdiffTsProdOutMax=[]  NTsProdOutMin=[]  NTsProdOutMax=[]  UintegralTsProdOutMin=[]  UintegralTsProdOutMax=[]  UngainTsProdOutMin=[]  UngainTsProdOutMax=[]  IntegratorContinuousStateAttributes=''  IntegratorStateMustResolveToSignalObject=off  IntegratorRTWStateStorageClass=Auto  FilterContinuousStateAttributes=''  FilterStateMustResolveToSignalObject=off  FilterRTWStateStorageClass=Auto  ParallelPVariant=InternalParameters  IdealPVariant=Disabled  IVariant=Disabled  DVariant=Disabled  IntegratorVariant=Disabled  SatVariant=Disabled  AWVariant=Disabled  PCopyVariant=Disabled  TRVariant=Disabled  FdbkBlocksVariant=Forward  IdealPFdbkVariant=Disabled  SatFdbkVariant=Disabled  DerivativeFilterVariant=Disabled  NVariant=Disabled  NCopyVariant=Disabled_SignalSpec  FilterICVariant=Disabled  IntegratorICVariant=Disabled  ExternalResetVariant=Disabled  TRSumVariant=Passthrough  SumFdbkVariant=Disabled  SumVariant=Passthrough_P  TsampFilterVariant=InternalTs  TsampNgainVariant=Passthrough  TsampIntegralVariant=Disabled_SignalSpec
  Radians to Degrees : simulink_extras/Transformations/Radians to Degrees
  Scope : Scope  NumInputPorts=4
  Scope1 : Scope  NumInputPorts=2
  Successive Linearizer2 : MATLAB Function  TreatAsAtomicUnit=on
  Switch1 : Switch  Criteria=u2 > Threshold  Threshold=25
  Switch2 : Switch  Criteria=u2 ~= 0
  Unary Minus : UnaryMinus
  front slip angle lookup table1 : simulink/Lookup Tables/Lookup Table Dynamic  LookUpMeth=Interpolation-Use End Values  OutDataType=fixdt('double')  OutScaling=[]  OutputDataTypeScalingMode=Specify via dialog  OutDataTypeStr=double  DoSatur=off
  tire linear region in front slip angle1 : Constant  Value=SlipAngle1
  Steering Angle : Outport
  ISB Fwf : Outport  Port=2
  ISB Fwr : Outport  Port=3
  wires:
  front slip angle lookup table1/1 -> Mapped into steering angle1/3(alphaf)
  Successive Linearizer2/6(Y) -> Bus Creator2/6
  Memory2/1 -> Successive Linearizer2/2(moves)
  Switch1/1 -> Scope1/1, MATLAB Function4/1(detection)  "detection"
  "If ISB is disenabled, compensator is off"/1 -> MATLAB Function3/2(Fxnet)
  [ref] -> Adaptive MPC Controller2/3
  Front lateral force1/1 -> front slip angle lookup table1/2
  [xdot] -> Scope/4, MATLAB Function4/2(Vx)  "vx"
  Successive Linearizer2/7(X) -> Bus Creator2/7
  [x] -> Mapped into steering angle1/1(x)
  [ks] -> Successive Linearizer2/4(ks)
  Successive Linearizer2/4(D) -> Bus Creator2/4
  Add1/1 -> PID Controller/1
  tire linear region in front slip angle1/1 -> front slip angle lookup table1/3
  [v_set] -> Add1/1
  [x] -> Successive Linearizer2/1(xk)
  Successive Linearizer2/5(U) -> Bus Creator2/5
  Demux1/1 -> front slip angle lookup table1/1  "Fyf"
  Successive Linearizer2/3(C) -> Bus Creator2/3
  Demux1/2 -> MATLAB Function3/1(Mx), Scope/1  "Mx"
  Bus Creator2/1 -> Adaptive MPC Controller2/1
  [xdot] -> Successive Linearizer2/3(Vx)
  Successive Linearizer2/9(DK) -> Adaptive MPC Controller2/4
  Adaptive MPC Controller2/1 -> Demux1/1
  [xdot] -> Add1/2
  MATLAB Function4/1(ymin) -> Adaptive MPC Controller2/5
  Adaptive MPC Controller2/2 -> Memory2/1
  Successive Linearizer2/2(B) -> Bus Creator2/2
  Successive Linearizer2/1(A) -> Bus Creator2/1
  Successive Linearizer2/8(DX) -> Bus Creator2/8
  MATLAB Function4/2(ymax) -> Adaptive MPC Controller2/6
  [xdot] -> Mapped into steering angle1/2(Vx)
  [x] -> MATLAB Function4/3(x)
  [x] -> Scope/3, Adaptive MPC Controller2/2  "states"
  states/1 -> [x]
  reference/1 -> [ref]
  v_set/1 -> [v_set]
  Vx/1 -> [xdot]
  curveture/1 -> [ks]
  Relative Distance/1 -> Scope1/2, Switch1/2  "distance"
  Constant/1 -> Switch1/1
  Constant1/1 -> Switch1/3
  Switch2/1 -> "If ISB is disenabled, compensator is off"/2, Adaptive MPC Controller2/7
  Radians to Degrees/1 -> Scope/2  "steering angle"
  Mapped into steering angle1/1(SteeringAngle) -> Unary Minus/1, Radians to Degrees/1
  MATLAB Function3/2(Fwr) -> ISB Fwr/1
  MATLAB Function3/1(Fwf) -> ISB Fwf/1
  Unary Minus/1 -> Steering Angle/1
  Gain/1 -> Add/2
  PID Controller/1 -> Add/1  "k(xdot_desired-xdot)"
  Constant2/1 -> Gain/1
  Switch/1 -> Switch2/2
  Constant3/1 -> Switch2/1
  Constant4/1 -> Switch2/3
  Add/1 -> "If ISB is disenabled, compensator is off"/1
  Constant5/1 -> "If ISB is disenabled, compensator is off"/3

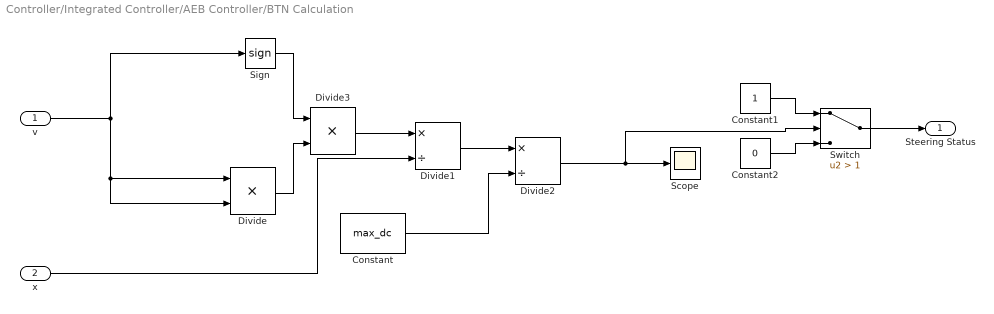
== system Controller/Integrated Controller/AEB Controller/BTN Calculation ==
  v : Inport
  x : Inport  Port=2
  Constant : Constant  Value=max_dc
  Constant1 : Constant
  Constant2 : Constant  Value=0
  Divide : Product  Inputs=**
  Divide1 : Product  Inputs=*/
  Divide2 : Product  Inputs=*/
  Divide3 : Product  Inputs=**
  Scope : Scope
  Sign : Signum
  Switch : Switch  Criteria=u2 > Threshold  Threshold=1
  Steering Status : Outport
  wires:
  Sign/1 -> Divide3/1
  Divide3/1 -> Divide1/1
  Divide2/1 -> Switch/2, Scope/1
  Constant1/1 -> Switch/1
  Constant2/1 -> Switch/3
  Switch/1 -> Steering Status/1
  Constant/1 -> Divide2/2
  Divide1/1 -> Divide2/1
  x/1 -> Divide1/2
  Divide/1 -> Divide3/2
  v/1 -> Divide/2, Divide/1, Sign/1

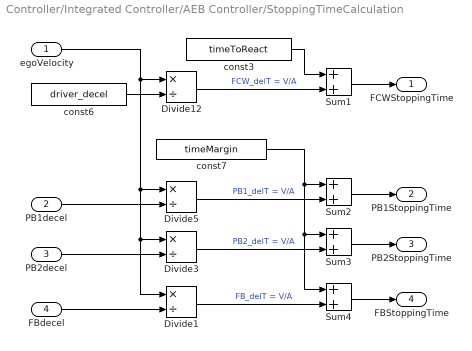
== system Controller/Integrated Controller/AEB Controller/StoppingTimeCalculation ==
  egoVelocity : Inport
  PB1decel : Inport  Port=2
  PB2decel : Inport  Port=3
  FBdecel : Inport  Port=4
  Divide{1,3,5,12} (4 alike) : Product  Inputs=*/
  Sum{1..4} (4 alike) : Sum
  const3 : Constant  Value=timeToReact  SampleTime=-1
  const6 : Constant  Value=driver_decel  SampleTime=-1
  const7 : Constant  Value=timeMargin  SampleTime=-1
  FCWStoppingTime : Outport  VectorParamsAs1DForOutWhenUnconnected=off
  PB1StoppingTime : Outport  Port=2  VectorParamsAs1DForOutWhenUnconnected=off
  PB2StoppingTime : Outport  Port=3  VectorParamsAs1DForOutWhenUnconnected=off
  FBStoppingTime : Outport  Port=4  VectorParamsAs1DForOutWhenUnconnected=off
  wires:
  Sum1/1 -> FCWStoppingTime/1
  Sum2/1 -> PB1StoppingTime/1
  Sum3/1 -> PB2StoppingTime/1
  Sum4/1 -> FBStoppingTime/1
  const7/1 -> Sum2/1, Sum4/1, Sum3/1
  egoVelocity/1 -> Divide1/1, Divide3/1, Divide5/1, Divide12/1
  Divide5/1 -> Sum2/2  "PB1_delT = V/A"
  Divide3/1 -> Sum3/2  "PB2_delT = V/A"
  Divide1/1 -> Sum4/2  "FB_delT = V/A"
  const6/1 -> Divide12/2
  PB1decel/1 -> Divide5/2
  PB2decel/1 -> Divide3/2
  FBdecel/1 -> Divide1/2
  const3/1 -> Sum1/1
  Divide12/1 -> Sum1/2  "FCW_delT = V/A"

== system Controller/Integrated Controller/AEB Controller/TTCCalculation ==
  mioDistance : Inport
  mioVelocity : Inport  Port=2
  Abs : Abs
  Divide11 : Product  Inputs=**
  Divide3 : Product  Inputs=*/
  Saturation : Saturate  UpperLimit=100  LowerLimit=0.01
  Sign : Signum
  Sum : Sum  Inputs=+-
  const1 : Constant  Value=headwayOffset  SampleTime=-1
  TTC : Outport  VectorParamsAs1DForOutWhenUnconnected=off
  wires:
  mioVelocity/1 -> Sign/1, Abs/1
  mioDistance/1 -> Sum/1
  Divide3/1 -> Divide11/1  "TTC"
  const1/1 -> Sum/2
  Sum/1 -> Divide3/1  "headway"
  Abs/1 -> Saturation/1
  Saturation/1 -> Divide3/2
  Sign/1 -> Divide11/2
  Divide11/1 -> TTC/1

== matlab function Controller/Tracking and Sensor Fusion/Find Rear Car ==
  data: confirmedTracks input; x output size=[1 1]; vx output size=[1 1]; lane input; mioTrackIndex output; positionSelector input
function [x,vx,mioTrackIndex] = findRearCar(confirmedTracks, lane, positionSelector)
% This function finds the lead car: a car in front of the ego car that
% satisfies all the criteria below:
% * Within the ego car's lane.
% * In front of the ego car.
% * Closest to the ego car.

% Note: If you change state definition, change the following:
%       State = [x;vx;y;vy;z;vz] (3D constant velocity)
numStates = 6;

% Initialize outputs and parameters
minX = cast(-1000, 'like', confirmedTracks.Tracks(1).State);  % Far enough forward so that no track is expected to exceed this distance
mioTrackIndex = 0;

% If lane detection is not available, the ego car is assumed to be located
% in the middle of its lane. The lane width is assumed to be 3.6m, typical
% highway lane width.
laneWidth = 3.6;
halfLaneWidth = laneWidth/2;

if lane.Left.Strength > 0.01
    lb = [lane.Left.CurvatureDerivative/6,...
        lane.Left.Curvature/2,...
        lane.Left.HeadingAngle,...
        lane.Left.LateralOffset];
else
    lb = single([0,0,0,halfLaneWidth]);
end

if lane.Right.Strength > 0.01
    rb = [lane.Right.CurvatureDerivative/6,...
        lane.Right.Curvature/2,...
        lane.Right.HeadingAngle,...
        lane.Right.LateralOffset];
else
    rb = single([0,0,0,-halfLaneWidth]);    
end

for i = 1:confirmedTracks.NumTracks
    position = positionSelector * confirmedTracks.Tracks(i).State;
    x = position(1); % Longitudinal position of the track relative to ego
    y = position(2); % Lateral position of the track relative to ego
    
    if x > minX && x < 0 % No point checking otherwise

        yleftLane  = polyval(lb,x); % lateral position of left lane
        yrightLane = polyval(rb,x); % lateral position of right lane
        
        % Find a new lead car
        if (yrightLane <= y) && (y <= yleftLane)
            minX = x;
            mioTrackIndex(:) = i;
        end
    end
end

if mioTrackIndex>0
    mioState = confirmedTracks.Tracks(mioTrackIndex).State;
else
    mioState = inf(numStates,1,'like',confirmedTracks.Tracks(1).State);
end

% Output:
x = mioState(1);    % Longitudinal position of the lead car
vx = mioState(2);   % Longitudinal velocity of the lead car

== stateflow chart Controller/Integrated Controller/AEB Controller/BrakingLogic ==
  state Default
    entry: BrakeStatus = 0;
    decel = 0;
  state FCW
    entry: BrakeStatus = 0;
    decel = 0;
  state Partial_Braking1
    entry: BrakeStatus = 1;
    decel = PB1decel;
  state Full_Braking
    entry: BrakeStatus = 3;
    decel = FBdecel;
  state Partial_Braking2
    entry: BrakeStatus = 2;
    decel = PB2decel;
  (default) -> Default
  Default -> (junction 114) [order 2]
  (junction 114) -> Full_Braking : [relativeDistance < default_spacing&&Vx>1]
  (junction 95) -> Default
  Full_Braking -> (junction 95) : [(stop==1) && TTC>0 && relativeDistance > default_spacing ]
  (junction 101) -> Default
  (junction 103) -> (junction 101) : [stop==1]
  (junction 97) -> Default
  (junction 99) -> (junction 97) : [stop==1]
  Default -> FCW [order 1] : [(abs(TTC)<FCWtime) && TTC<0]
  FCW -> Default [order 2] : [abs(TTC)>=1.2*FCWtime]
  FCW -> Partial_Braking1 [order 1] : [(abs(TTC) < PB1time) && TTC<0]
  Partial_Braking1 -> (junction 99) [order 1]
  Partial_Braking1 -> Partial_Braking2 [order 2] : [(abs(TTC) < PB2time) && TTC<0]
  Partial_Braking2 -> (junction 103) [order 2]
  Partial_Braking2 -> Full_Braking [order 1] : [(abs(TTC) < FBtime) && TTC<0]
  data: relativeDistance input; TTC input; FCWtime input; PB1time input; PB2time input; FBtime input; PB1decel input; PB2decel input; FBdecel input; BrakeStatus output; decel output; stop input; default_spacing parameter; Vx input

== matlab function Controller/Integrated Controller/MATLAB Function ==
  data: acc1 input; acc output; acc2 input; theta1 input; theta2 input; brake input; steer input; theta output; xdot input
function [acc,theta] = fcn(acc1,acc2,theta1,theta2,brake,steer,xdot)

if steer == 0
    if brake ~= 0
    acc = acc2;
    else
        if xdot<=0
            acc = 0;
        else
            acc = acc1;
        end
    end
    theta = theta1;
else
    theta = theta2;
    acc = 0;
end

%(1) test steering controller
% theta = theta2;
% acc = 0;

== matlab function Controller/Tracking and Sensor Fusion/Find Lead Car ==
  data: confirmedTracks input; x output size=[1 1]; vx output size=[1 1]; lane input; mioTrackIndex output; positionSelector input
function [x,vx,mioTrackIndex] = findLeadCar(confirmedTracks, lane, positionSelector)
% This function finds the lead car: a car in front of the ego car that
% satisfies all the criteria below:
% * Within the ego car's lane.
% * In front of the ego car.
% * Closest to the ego car.

% Note: If you change state definition, change the following:
%       State = [x;vx;y;vy;z;vz] (3D constant velocity)
numStates = 6;

% Initialize outputs and parameters
maxX = cast(1000, 'like', confirmedTracks.Tracks(1).State);  % Far enough forward so that no track is expected to exceed this distance
mioTrackIndex = 0;

% If lane detection is not available, the ego car is assumed to be located
% in the middle of its lane. The lane width is assumed to be 3.6m, typical
% highway lane width.
laneWidth = 3.6;
halfLaneWidth = laneWidth/2;

if lane.Left.Strength > 0.01
    lb = [lane.Left.CurvatureDerivative/6,...
        lane.Left.Curvature/2,...
        lane.Left.HeadingAngle,...
        lane.Left.LateralOffset];
else
    lb = single([0,0,0,halfLaneWidth]);
end

if lane.Right.Strength > 0.01
    rb = [lane.Right.CurvatureDerivative/6,...
        lane.Right.Curvature/2,...
        lane.Right.HeadingAngle,...
        lane.Right.LateralOffset];
else
    rb = single([0,0,0,-halfLaneWidth]);    
end

for i = 1:confirmedTracks.NumTracks
    position = positionSelector * confirmedTracks.Tracks(i).State;
    x = position(1); % Longitudinal position of the track relative to ego
    y = position(2); % Lateral position of the track relative to ego
    
    if x < maxX && x > 0 % No point checking otherwise

        yleftLane  = polyval(lb,x); % lateral position of left lane
        yrightLane = polyval(rb,x); % lateral position of right lane
        
        % Find a new lead car
        if (yrightLane <= y) && (y <= yleftLane)
            maxX = x;
            mioTrackIndex(:) = i;
        end
    end
end

if mioTrackIndex>0
    mioState = confirmedTracks.Tracks(mioTrackIndex).State;
else
    mioState = inf(numStates,1,'like',confirmedTracks.Tracks(1).State);
end

% Output:
x = mioState(1);    % Longitudinal position of the lead car
vx = mioState(2);   % Longitudinal velocity of the lead car

== matlab function Controller/Estimate Lane Center/MATLAB Function ==
  data: lanes input
  events: fcnLeftAndRight output FUNCTION_CALL_EVENT; fcnLeftOnly output FUNCTION_CALL_EVENT; fcnRightOnly output FUNCTION_CALL_EVENT; fcnNone output FUNCTION_CALL_EVENT
function fcn(lanes)

leftStrength  = lanes.Left.Strength;
rightStrength = lanes.Right.Strength;

if (leftStrength > 0) && (rightStrength > 0)
   fcnLeftAndRight();
   
elseif leftStrength > 0
    fcnLeftOnly();
    
elseif rightStrength > 0
    fcnRightOnly();
    
else
    fcnNone();
end

== matlab function Controller/Integrated Controller/Integrated Steering Controller/MATLAB Function3 ==
  data: Fwf output size=[2,1]; Mx input; Fwr output size=[2,1]; Fxnet input
function [Fwf,Fwr] = fcn(Mx,Fxnet)

w = 1.4; % the width of the car

Fwf = zeros(2,1);
Fwr = zeros(2,1);

if Mx > 0
    Fwf(1) = Fxnet/2-Mx/w;
    Fwf(2) = Fxnet/2+0;
    Fwr(1) = 0-Mx/w;
    Fwr(2) = 0;
elseif Mx < 0
    Fwf(1) = Fxnet/2+0;
    Fwf(2) = Fxnet/2+Mx/w;
    Fwr(1) = 0;
    Fwr(2) = 0+Mx/w;
else
    Fwf(1) = Fxnet/2+0;
    Fwf(2) = Fxnet/2+0;
    Fwr(1) = 0;
    Fwr(2) = 0;
end

== matlab function Controller/Integrated Controller/Integrated Steering Controller/MATLAB Function4 ==
  data: detection input; ymin output; ymax output; Vx input; x input
function [ymin,ymax] = fcn(detection,Vx,x)

miu = 0.7; %frction cooeficient 0.7 for dry road and 0.4 for wet
g = 9.81; % gravity
m = 2272;   %mass
lf = 1.11;  % distance from front axle to the mass center
lr = 1.67;  % distance from rear axle to the mass center
C_a = 1.3e5; % rear cornering stifness

Fz = m*g*lf/(lf+lr)/2; % the load that beared by the rear tire

rmax = g*miu/Vx; %max yaw rate
threshold = atan(3*miu*Fz/C_a);

r = x(2);
vmax = lr*r+Vx*threshold;   %max lateral velocity
vmin = lr*r-Vx*threshold;   %min lateral velocity

if detection == 1
    ymin = [vmin -rmax -pi/2 5]';%-5 means 5 in world coordinate (steering left)
    ymax = [vmax rmax pi/2 10]';
else
    ymin = [vmin -rmax -pi/2 -10]';
    ymax = [vmax rmax pi/2 10]';
end

== matlab function Controller/Integrated Controller/Integrated Steering Controller/Mapped into steering angle1 ==
  data: x input; Vx input; alphaf input; SteeringAngle output
function SteeringAngle = fcn(x,Vx, alphaf)

lf = 1.11;  % distance from front axle to the mass center

Vy = x(1); %lateral velocity
r = x(2);  %yaw rate
SteeringAngle = Vy/Vx+lf*r/Vx-alphaf;
